simulink model "TrajectoryControl"  (R2022b)
settings: Solver=FixedStepAuto  StartTime=0.0  StopTime=30  FixedStep=0.001  RelTol=1e-3
undefined symbols (not defined in the file): h, headingangle, km, m, s, smiData, X, x, Y, Z
libraries: sm_lib x213, aerolibconvert2 x17, simulink_extras x15, nesl_utility x14, autolibshared x3, slpidlib x1, vehdynlibsteering x1, autolibutils x1
(part 1 of 5)
settings Model: Creator=dangm  LastModifiedBy=ASUS
settings SolverCC: ZeroCrossAlgorithm=Adaptive  AlgebraicLoopSolver=LineSearch
settings DebuggingCC: IgnoredZcDiagnostic=none  UnconnectedInputMsg=warning  UnconnectedOutputMsg=warning  UnconnectedLineMsg=warning  SFMachineParentedDataDiag=warning
settings ModelReferenceCC: EnableRefExpFcnMdlSchedulingChecks=on
settings ExplorerConfigSet: InternalSimMechanicsExplorerSettings="<ExplorerConfiguration><canonicalview>planar_xy</canonicalview><AnimationSetting><BasePlaybackSpeed>1.0</BasePlaybackSpeed><PlaybackSpeedFactor>1.0</PlaybackSpeedFactor></AnimationSetting><TilePanel><TileInfo><Tiles Columns=\"1\" Count=\"1\" Rows=\"1\"><Column Weight=\"1\"/><Row Weight=\"1\"/><Tile Height=\"1\" Width=\"1\" X=\"0\" Y=\"0\"/></Tiles></TileInfo><SceneInfo><SceneViewer><BGColor><R>0.60000002384185791</R><G>0.60000002384185791</G><B>0.60000002384185791</B></BGColor><Camera><DoPerspective>off</DoPerspective><Position><X>1.38151927744802361</X><Y>-0.113937833645223696</Y><Z>-0.183681847979671575</Z></Position><Center><X>0.0576620377884289326</X><Y>0.060665039066758325</Y><Z>0.733764197719871003</Z></Center><Up><X>0.27535581417737931</X><Y>0.936019488942585909</Y><Z>0.219195556338108416</Z></Up><ViewLimDist>1</ViewLimDist><YLim>0.747285369634628327</YLim><XLim>1.35610315607225207</XLim></Camera></SceneViewer></SceneInfo></TilePanel><MechEditorPanel><Cameras/><GfxPanelCameraMap/><VideoCreator><PlaybackSpeedRatio>1.0</PlaybackSpeedRatio><FrameRate>30</FrameRate><VideoFormat>Motion JPEG AVI</VideoFormat><FrameSize>auto</FrameSize></VideoCreator></MechEditorPanel></ExplorerConfiguration>"

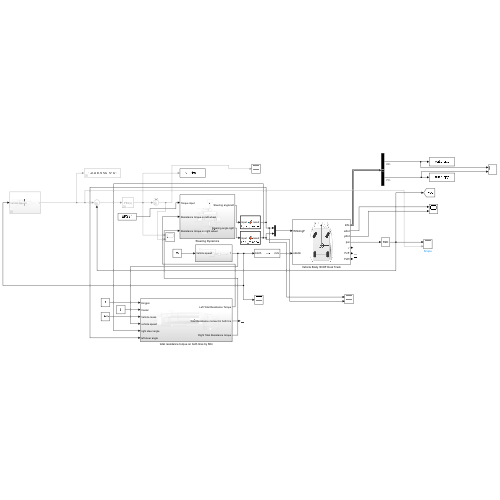
[thumbnail: Simulink's stored preview of the top-level diagram]
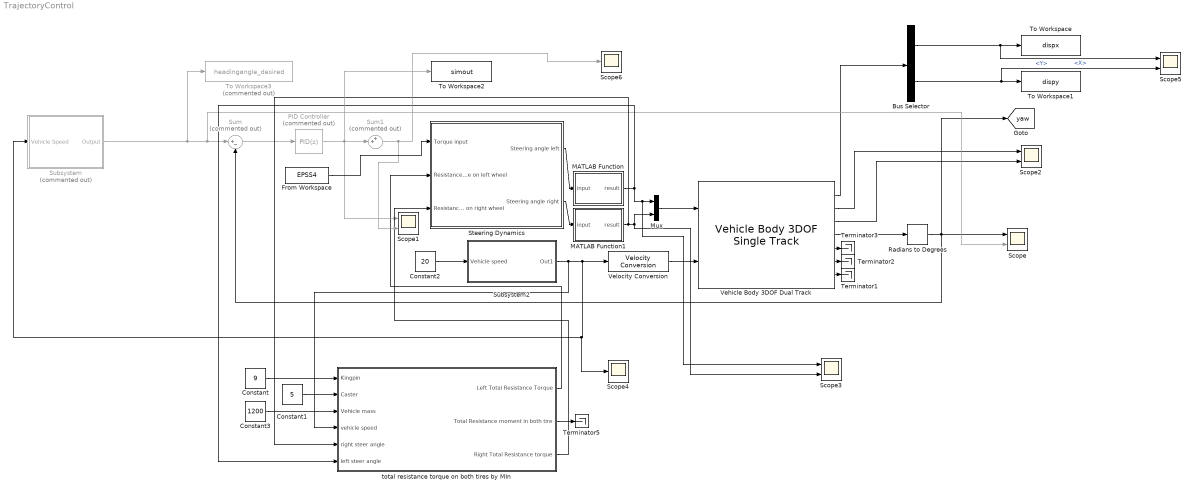
== system TrajectoryControl ==
  Bus Selector : BusSelector  OutputSignals=InertFrm.Cg.Disp.X,InertFrm.Cg.Disp.Y
  Constant : Constant  Value=9
  Constant1 : Constant  Value=5
  Constant2 : Constant  Value=20
  Constant3 : Constant  Value=1200
  From Workspace : FromWorkspace  VariableName=EPSS4
  MATLAB Function : MATLAB Function  TreatAsAtomicUnit=on
  MATLAB Function1 : MATLAB Function  TreatAsAtomicUnit=on
  Mux : Mux  Inputs=2
  PID Controller : slpidlib/PID Controller  Commented=on  Controller=PID  Form=Parallel  TimeDomain=Discrete-time  UseExternalTs=off  SampleTime=-1  IntegratorMethod=Forward Euler  FilterMethod=Forward Euler  ControllerParametersSource=internal  P=1  I=0  UseKiTs=off  D=20  N=205.123568338568  UseFilter=off  TunerSelectOption=Transfer Function Based (PID Tuner App)  InitialConditionSource=internal  InitialConditionForIntegrator=0  InitialConditionForFilter=0  DifferentiatorICPrevScaledInput=0  ExternalReset=none  TrackingMode=off  Kt=1  LimitOutput=off  SatLimitsSource=internal  UpperSaturationLimit=0  LowerSaturationLimit=-10  LinearizeAsGain=on  AntiWindupMode=none  Kb=1  LimitIntegrator=off  UpperIntegratorSaturationLimit=inf  LowerIntegratorSaturationLimit=-inf  POutMin=[]  POutMax=[]  IOutMin=[]  IOutMax=[]  DOutMin=[]  DOutMax=[]  NOutMin=[]  NOutMax=[]  SumOutMin=[]  SumOutMax=[]  SaturationOutMin=[]  SaturationOutMax=[]  PParamMin=[]  PParamMax=[]  IParamMin=[]  IParamMax=[]  DParamMin=[]  DParamMax=[]  NParamMin=[]  NParamMax=[]  KbParamMin=[]  KbParamMax=[]  KtParamMin=[]  KtParamMax=[]  KbOutMin=[]  KbOutMax=[]  KtOutMin=[]  KtOutMax=[]  IntegratorOutMin=[]  IntegratorOutMax=[]  FilterOutMin=[]  FilterOutMax=[]  SumI1OutMin=[]  SumI1OutMax=[]  SumI2OutMin=[]  SumI2OutMax=[]  SumI3OutMin=[]  SumI3OutMax=[]  SumI4OutMin=[]  SumI4OutMax=[]  SumDOutMin=[]  SumDOutMax=[]  DifferentiatorOutMin=[]  DifferentiatorOutMax=[]  FilterDiffOutCoefMin=[]  FilterDiffOutCoefMax=[]  ReciprocalOutMin=[]  ReciprocalOutMax=[]  SumDenOutMin=[]  SumDenOutMax=[]  SumNumOutMin=[]  SumNumOutMax=[]  DivideOutMin=[]  DivideOutMax=[]  UdiffTsProdOutMin=[]  UdiffTsProdOutMax=[]  NTsProdOutMin=[]  NTsProdOutMax=[]  UintegralTsProdOutMin=[]  UintegralTsProdOutMax=[]  UngainTsProdOutMin=[]  UngainTsProdOutMax=[]  ClampingZeroOutDataTypeStr=Inherit: Inherit via back propagation  ClampingZeroOutMin=[]  ClampingZeroOutMax=[]  FilterDenConstantOutDataTypeStr=Inherit: Inherit via back propagation  FilterDenConstantOutMin=[]  FilterDenConstantOutMax=[]  PCopyOutDataTypeStr=Inherit: Inherit via back propagation  PCopyOutMin=[]  PCopyOutMax=[]  NCopyOutDataTypeStr=Inherit: Inherit via back propagation  NCopyOutMin=[]  NCopyOutMax=[]  IntegratorContinuousStateAttributes=''  IntegratorStateMustResolveToSignalObject=off  IntegratorRTWStateStorageClass=Auto  FilterContinuousStateAttributes=''  FilterStateMustResolveToSignalObject=off  FilterRTWStateStorageClass=Auto  ParallelPVariant=InternalParameters  IdealPVariant=Disabled  IVariant=InternalParameters  DVariant=InternalParameters  IntegratorVariant=Discrete  SatVariant=Disabled  AWVariant=Passthrough  PCopyVariant=Disabled  TRVariant=Disabled  FdbkBlocksVariant=Forward  IdealPFdbkVariant=Disabled  SatFdbkVariant=Disabled  DerivativeFilterVariant=Differentiator  NVariant=Passthrough  NCopyVariant=Disabled_SignalSpec  FilterICVariant=InternalICsDifferentiator  IntegratorICVariant=InternalICs  ExternalResetVariant=Disabled  TRSumVariant=Passthrough  SumFdbkVariant=Disabled  SumVariant=Sum_PID  TsampFilterVariant=InternalTs  TsampNgainVariant=Passthrough  TsampIntegralVariant=Passthrough  ExternalSaturationOutDataTypeStr=Inherit: Same as second input
  Radians to Degrees : simulink_extras/Transformations/Radians to Degrees
  Scope{,1..3,5} (5 alike) : Scope  NumInputPorts=2
  Scope4 : Scope
  Scope6 : Scope
  Steering Dynamics : Subsystem
  Subsystem : Subsystem  Commented=on
  Subsystem2 : Subsystem
  Sum : Sum  Commented=on  Inputs=|+-
  Sum1 : Sum  Commented=on  Inputs=++|
  Terminator{1..3,5} (4 alike) : Terminator
  To Workspace : ToWorkspace  VariableName=dispx  SaveFormat=Structure With Time  SampleTime=-1
  To Workspace1 : ToWorkspace  VariableName=dispy  SaveFormat=Structure With Time  SampleTime=-1
  To Workspace2 : ToWorkspace  VariableName=simout  SaveFormat=Structure With Time  SampleTime=-1
  To Workspace3 : ToWorkspace  Commented=on  VariableName=headingangle_desired  SaveFormat=Structure With Time  SampleTime=-1
  Vehicle Body 3DOF Dual Track : autolibshared/Vehicle Body 3DOF Single Track  trackMode=Dual  inputMode=External longitudinal velocity  frontSteerMode=on  rearSteerMode=off  windMode=off  muMode=off  extFMode=off  extMMode=off  htchFMode=off  htchMMode=off  extXo=off  extpsio=off  extxdoto=off  extro=off  extYo=off  extTamb=off  extydoto=off  aMode=2  NF=2  NR=2  m=2000  a=1.4  b=1.6  h=0.35  dh=1  hh=0.2  X_o=0  xdot_o=0  CalphaMode=off  sigmaMode=on  d=0  hl=0  w=[1.4,1.4]  Cy_f=12e3  Cy_r=11e3  sigma_f=.1  sigma_r=.1  alpha_f_brk=[-.1 .1]  Cy_f_data=[-9e3 9e3]  alpha_r_brk=[-.1 .1]  Cy_r_data=[-9e3 9e3]  Y_o=0  ydot_o=0  Izz=4000  psi_o=0  r_o=0  Af=2  Cd=.3  Cl=.1  Cpm=.1  beta_w=[0:0.01:0.3]  Cs=[0:0.03:0.9]  Cym=[0:0.01:0.3]  Pabs=101325  Tair=273  g=9.81  mu=1  xdot_tol=.01  Fznom=5000  Fxtire_sat=7e4  Fytire_sat=7e4  longOff=0  latOff=0  vertOff=0  wrapAng=off
  Velocity Conversion : aerolibconvert2/Velocity Conversion  IU=km/h  OU=m/s
  total resistance torque on both tires by MIn : Subsystem
  tag scope: yaw=global
  wires:
  Mux/1 -> Vehicle Body 3DOF Dual Track/1
  Vehicle Body 3DOF Dual Track/7 -> Terminator1/1
  Vehicle Body 3DOF Dual Track/6 -> Terminator2/1
  Vehicle Body 3DOF Dual Track/5 -> Terminator3/1
  Vehicle Body 3DOF Dual Track/1 -> Bus Selector/1
  Vehicle Body 3DOF Dual Track/3 -> Scope2/2
  Vehicle Body 3DOF Dual Track/4 -> Radians to Degrees/1
  Radians to Degrees/1 -> [yaw], Scope/1, Sum/2
  Bus Selector/1 -> Scope5/1, To Workspace/1  "<X>"
  Bus Selector/2 -> Scope5/2, To Workspace1/1  "<Y>"
  Velocity Conversion/1 -> Vehicle Body 3DOF Dual Track/2
  Vehicle Body 3DOF Dual Track/2 -> Scope2/1
  Sum/1 -> PID Controller/1
  total resistance torque on both tires by MIn/1(Left Total Resistance Torque) -> Steering Dynamics/2(Resistance torque on left wheel)
  Subsystem2/1(Out1) -> total resistance torque on both tires by MIn/4("vehicle speed "), Scope4/1, Subsystem/1("Vehicle Speed "), Velocity Conversion/1
  Constant2/1 -> Subsystem2/1(Vehicle speed)
  Subsystem/1(Output) -> To Workspace3/1, Scope/2, Sum/1
  Steering Dynamics/1(Steering angle left) -> MATLAB Function/1(input)
  MATLAB Function/1(result) -> total resistance torque on both tires by MIn/6(left steer angle), Scope3/1, Mux/1
  Steering Dynamics/2(Steering angle right) -> MATLAB Function1/1(input)
  MATLAB Function1/1(result) -> total resistance torque on both tires by MIn/5(right steer angle), Mux/2, Scope3/2
  PID Controller/1 -> Sum1/2, To Workspace2/1, Scope1/1
  total resistance torque on both tires by MIn/3(Right Total Resistance torque) -> Steering Dynamics/3(Resistance torque on right wheel)
  total resistance torque on both tires by MIn/2(Total Resistance moment in both tire) -> Terminator5/1
  Constant/1 -> total resistance torque on both tires by MIn/1(Kingpin)
  Constant1/1 -> total resistance torque on both tires by MIn/2(Caster)
  Constant3/1 -> total resistance torque on both tires by MIn/3(Vehicle mass)
  Sum1/1 -> Scope1/2, Scope6/1
  From Workspace/1 -> Steering Dynamics/1(Torque input)

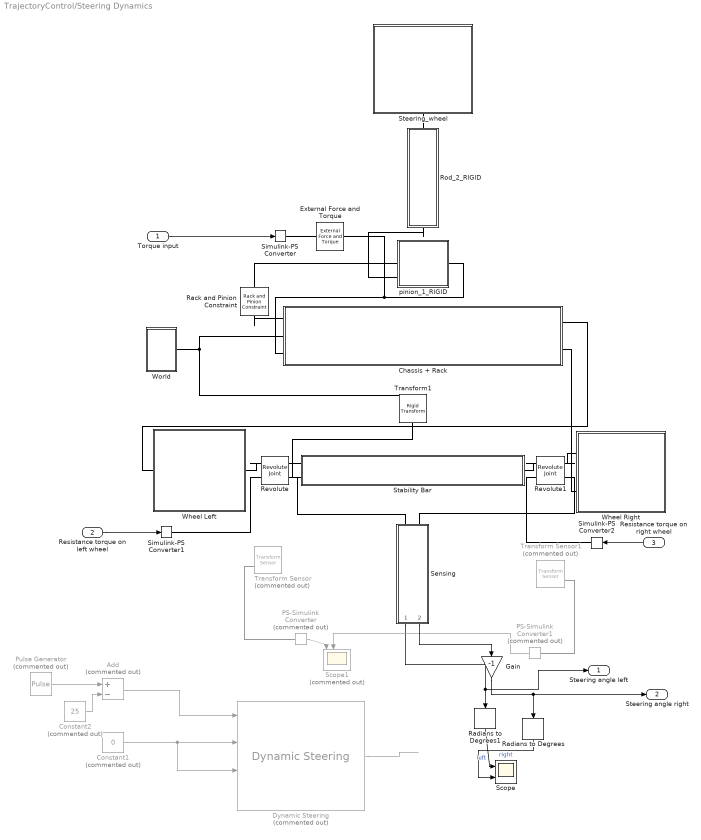
== system TrajectoryControl/Steering Dynamics ==
  Torque input : Inport
  Resistance torque on left wheel : Inport  Port=2
  Resistance torque on right wheel : Inport  Port=3
  Add : Sum  Commented=on  Inputs=+-
  Chassis + Rack : Subsystem
      mask Display: image('E:\Hoc\do an\(final) download\test14\image\Chassis+rack.png'); % Use "Edit Image" on toolstrip to change.
  Constant1 : Constant  Commented=on  Value=0
  Constant2 : Constant  Commented=on  Value=25
  Dynamic Steering : vehdynlibsteering/Dynamic Steering  Commented=on  StrgType=Rack and pinion  StrgRatioType=Constant  PwrAst=off  Loc=Front  TrckWdth=1  WhlBase=1.524  StrgRng=1.25*pi  StrgAngBpts="[-6.2832   -5.0265   -3.7699   -2.5133   -1.2566         0    1.2566    2.5133    3.7699    5.0265    6.2832]"  StrgRatioTbl=|  StrgRatio=13.5  StrgArmLngth=0.1  RckCsLngth=0.5  TieRodLngth=0.248  D=0.2  PnnRadiusTbl="[0.0055    0.0055    0.0056    0.0057    0.0057    0.0057    0.0058    0.0057    0.0056    0.0055    0.0055]"  PnnRadius=0.0057  RodLngth=0.1  ParaArmLngth=0.9  J1=0.1  J2=0.01  beta_u=0.1  beta_l=0.1  b1=0.001  k1=30  b2=1  b3=0.001  theta_o=0  omega_o=0  FricTrq=0  TrqBpts=[-100 0 100]  VehSpdBpts=[0 20]  TrqTbl=[0 -100;0 0;0 100]  TrqLmt=100  PwrLmt=1000  Eta=1  omega_c=200  aMode=2
      | [13.5000   13.3750   13.2500   13.1250   13.0000   13.0000   13.0000   13.1250   13.2500   13.3750   13.5000
      | ]
  External Force and Torque : sm_lib/Forces and Torques/External Force and Torque  ForceResolutionFrame=AttachedFrame  EnableForceX=off  EnableForceY=off  EnableForceZ=off  EnableForce=off  TorqueResolutionFrame=AttachedFrame  EnableTorqueX=off  EnableTorqueY=off  EnableTorqueZ=on  EnableTorque=off
  Gain : Gain  Gain=-1
  PS-Simulink Converter : nesl_utility/PS-Simulink Converter  Commented=on  PhysicalDomain=network_engine_domain  SubClassName=ps_output  LeftPortType=input  RightPortType=output  PseudoPeriodic=off  Frequencies=[]  VectorFormat=1-D array  Unit=inherit  AffineConversion=off
  PS-Simulink Converter1 : nesl_utility/PS-Simulink Converter  Commented=on  PhysicalDomain=network_engine_domain  SubClassName=ps_output  LeftPortType=input  RightPortType=output  PseudoPeriodic=off  Frequencies=[]  VectorFormat=1-D array  Unit=inherit  AffineConversion=off
  Pulse Generator : DiscretePulseGenerator  Commented=on  PulseType=Time based  Amplitude=50  Period=10  PulseWidth=50
  Rack and Pinion Constraint : sm_lib/Gears and Couplings/Gears/Rack and Pinion Constraint  PinionRadius=30  PinionRadiusUnits=mm
  Radians to Degrees : simulink_extras/Transformations/Radians to Degrees
  Radians to Degrees1 : simulink_extras/Transformations/Radians to Degrees
  Revolute : sm_lib/Joints/Revolute Joint  JointMode=Normal  SenseConstraintForce=off  SenseConstraintForceX=off  SenseConstraintForceY=off  SenseConstraintForceZ=off  SenseConstraintTorque=off  SenseConstraintTorqueX=off  SenseConstraintTorqueY=off  SenseConstraintTorqueZ=off  SenseTotalForce=off  SenseTotalForceX=off  SenseTotalForceY=off  SenseTotalForceZ=off  SenseTotalTorque=off  SenseTotalTorqueX=off  SenseTotalTorqueY=off  SenseTotalTorqueZ=off  CompositeWrenchDir=FollowerOnBase  CompositeWrenchFrame=BaseFrame  EquilibriumPosition=0  EquilibriumPositionUnits=deg  SpringStiffness=0.0524  SpringStiffnessUnits=N*m/deg  DampingCoefficient=1.5  DampingCoefficientUnits=N*m/(deg/s)  TorqueActuationMode=InputTorque  MotionActuationMode=ComputedMotion  SensePosition=on  SenseVelocity=off  SenseAcceleration=off  SenseTorqueForce=off  SenseLowerLimitTorqueForce=off  SenseUpperLimitTorqueForce=off  LowerLimitSpecify=on  LowerLimitBound=-2  LowerLimitBoundUnits=rad  LowerLimitStiffness=1e4  LowerLimitStiffnessUnits=N*m/deg  LowerLimitDamping=100  LowerLimitDampingUnits=N*m/(deg/s)  LowerLimitTransitionRegionWidth=0.1  LowerLimitTransitionRegionWidthUnits=deg  UpperLimitSpecify=on  UpperLimitBound=-1  UpperLimitBoundUnits=rad  UpperLimitStiffness=1e4  UpperLimitStiffnessUnits=N*m/deg  UpperLimitDamping=100  UpperLimitDampingUnits=N*m/(deg/s)  UpperLimitTransitionRegionWidth=0.1  UpperLimitTransitionRegionWidthUnits=deg  PositionTargetSpecify=on  PositionTargetPriority=High  PositionTargetValue=-89.678329494  PositionTargetValueUnits=deg  VelocityTargetSpecify=on  VelocityTargetPriority=High  VelocityTargetValue=0  VelocityTargetValueUnits=deg/s
  Revolute1 : sm_lib/Joints/Revolute Joint  JointMode=Normal  SenseConstraintForce=off  SenseConstraintForceX=off  SenseConstraintForceY=off  SenseConstraintForceZ=off  SenseConstraintTorque=off  SenseConstraintTorqueX=off  SenseConstraintTorqueY=off  SenseConstraintTorqueZ=off  SenseTotalForce=off  SenseTotalForceX=off  SenseTotalForceY=off  SenseTotalForceZ=off  SenseTotalTorque=off  SenseTotalTorqueX=off  SenseTotalTorqueY=off  SenseTotalTorqueZ=off  CompositeWrenchDir=FollowerOnBase  CompositeWrenchFrame=BaseFrame  EquilibriumPosition=0  EquilibriumPositionUnits=deg  SpringStiffness=0.0524  SpringStiffnessUnits=N*m/deg  DampingCoefficient=1.5  DampingCoefficientUnits=N*m/(deg/s)  TorqueActuationMode=InputTorque  MotionActuationMode=ComputedMotion  SensePosition=on  SenseVelocity=off  SenseAcceleration=off  SenseTorqueForce=off  SenseLowerLimitTorqueForce=off  SenseUpperLimitTorqueForce=off  LowerLimitSpecify=on  LowerLimitBound=-2  LowerLimitBoundUnits=rad  LowerLimitStiffness=1e4  LowerLimitStiffnessUnits=N*m/deg  LowerLimitDamping=100  LowerLimitDampingUnits=N*m/(deg/s)  LowerLimitTransitionRegionWidth=0.1  LowerLimitTransitionRegionWidthUnits=deg  UpperLimitSpecify=on  UpperLimitBound=-1  UpperLimitBoundUnits=rad  UpperLimitStiffness=1e4  UpperLimitStiffnessUnits=N*m/deg  UpperLimitDamping=100  UpperLimitDampingUnits=N*m/(deg/s)  UpperLimitTransitionRegionWidth=0.1  UpperLimitTransitionRegionWidthUnits=deg  PositionTargetSpecify=on  PositionTargetPriority=Low  PositionTargetValue=smiData.RevoluteJoint(2).Rz.Pos-2.7  PositionTargetValueUnits=deg  VelocityTargetSpecify=on  VelocityTargetPriority=High  VelocityTargetValue=0  VelocityTargetValueUnits=deg/s
  Rod_2_RIGID : Subsystem
      mask Display: image('rod.png'); % Use "Edit Image" on toolstrip to change.
  Scope : Scope  NumInputPorts=2
  Scope1 : Scope  Commented=on  NumInputPorts=4
  "Sensing " : Subsystem
  Simulink-PS Converter : nesl_utility/Simulink-PS Converter  PhysicalDomain=network_engine_domain  SubClassName=ps_input  LeftPortType=input  RightPortType=output  PseudoPeriodic=off  Frequencies=[]  NoiseDistribution=none  NoiseParameters=[]  Unit=N*m  AffineConversion=off  FilteringAndDerivatives=provide  SimscapeFilterOrder=1  InputFilterTimeConstant=0.001  UdotUserProvided=0
  Simulink-PS Converter1 : nesl_utility/Simulink-PS Converter  PhysicalDomain=network_engine_domain  SubClassName=ps_input  LeftPortType=input  RightPortType=output  PseudoPeriodic=off  Frequencies=[]  NoiseDistribution=none  NoiseParameters=[]  Unit=N*m  AffineConversion=off  FilteringAndDerivatives=provide  SimscapeFilterOrder=1  InputFilterTimeConstant=0.001  UdotUserProvided=0
  Simulink-PS Converter2 : nesl_utility/Simulink-PS Converter  PhysicalDomain=network_engine_domain  SubClassName=ps_input  LeftPortType=input  RightPortType=output  PseudoPeriodic=off  Frequencies=[]  NoiseDistribution=none  NoiseParameters=[]  Unit=N*m  AffineConversion=off  FilteringAndDerivatives=provide  SimscapeFilterOrder=2  InputFilterTimeConstant=0.001  UdotUserProvided=0
  Stability Bar : Subsystem
      mask Display: image('E:\Hoc\do an\(final) download\test14\image\stability bar.png'); % Use "Edit Image" on toolstrip to change.
  Steering_wheel : Subsystem
      mask Display: image('$imagefile'); % Use "Edit Image" on toolstrip to change.
  Transform Sensor : sm_lib/Frames and Transforms/Transform Sensor  Commented=on  MeasurementFrame=Base  SenseAngle=on  SenseAxis=off  SenseQ=off  SenseR=off  SenseRotationSequence=off  RotationSequence=XYX  SenseOmegaX=off  SenseOmegaY=off  SenseOmegaZ=off  SenseQDot=off  SenseRDot=off  SenseAlphaX=off  SenseAlphaY=off  SenseAlphaZ=off  SenseQDDot=off  SenseRDDot=off  SenseX=off  SenseY=off  SenseZ=off  SenseRad=off  SenseAzim=off  SenseDist=off  SenseInc=off  SenseXDot=off  SenseYDot=off  SenseZDot=off  SenseRadDot=off  SenseAzimDot=off  SenseDistDot=off  SenseIncDot=off  SenseXDDot=off  SenseYDDot=off  SenseZDDot=off  SenseRadDDot=off  SenseAzimDDot=off  SenseDistDDot=off  SenseIncDDot=off
  Transform Sensor1 : sm_lib/Frames and Transforms/Transform Sensor  Commented=on  MeasurementFrame=Base  SenseAngle=on  SenseAxis=off  SenseQ=off  SenseR=off  SenseRotationSequence=off  RotationSequence=XYX  SenseOmegaX=off  SenseOmegaY=off  SenseOmegaZ=off  SenseQDot=off  SenseRDot=off  SenseAlphaX=off  SenseAlphaY=off  SenseAlphaZ=off  SenseQDDot=off  SenseRDDot=off  SenseX=off  SenseY=off  SenseZ=off  SenseRad=off  SenseAzim=off  SenseDist=off  SenseInc=off  SenseXDot=off  SenseYDot=off  SenseZDot=off  SenseRadDot=off  SenseAzimDot=off  SenseDistDot=off  SenseIncDot=off  SenseXDDot=off  SenseYDDot=off  SenseZDDot=off  SenseRadDDot=off  SenseAzimDDot=off  SenseDistDDot=off  SenseIncDDot=off
  Transform1 : sm_lib/Frames and Transforms/Rigid Transform  TranslationMethod=Cartesian  TranslationStandardOffset=0  TranslationLengthUnit=mm  TranslationStandardAxis=+Z  TranslationCartesianOffset=smiData.RigidTransform(48).translation  TranslationROffset=0  TranslationROffsetUnits=m  TranslationZOffset=0  TranslationZOffsetUnits=m  TranslationThetaOffset=0  TranslationThetaOffsetUnits=deg  RotationMethod=ArbitraryAxis  RotationAngleUnits=rad  RotationStandardAxis=+Z  RotationAngle=smiData.RigidTransform(48).angle  RotationArbitraryAxis=smiData.RigidTransform(48).axis  FollAlignAxisA=+X  BaseAlignAxisA=+Y  FollAlignAxisB=+Y  BaseAlignAxisB=+Z  RotationSequenceAxes=FollowerAxes  RotationSequence=XYX  RotationSequenceAngles=[0 0 0]  RotationSequenceAnglesUnits=deg  RotationMatrix=[1 0 0; 0 1 0; 0 0 1]  Quaternion=[1 0 0 0]
  Wheel Left : Subsystem
      mask Display: image('E:\Hoc\do an\(final) download\test14\image\wheel.png'); % Use "Edit Image" on toolstrip to change.
  Wheel Right : Subsystem
      mask Display: image('E:\Hoc\do an\(final) download\test14\image\wheel.png'); % Use "Edit Image" on toolstrip to change.
  World : Subsystem
  pinion_1_RIGID : Subsystem
      mask Display: image('pinion.png'); % Use "Edit Image" on toolstrip to change.
  Steering angle left : Outport
  Steering angle right : Outport  Port=2
  wires:
  "Sensing "/1(Steering angle left (rad)) -> Steering angle left/1, Radians to Degrees1/1
  Add/1 -> Dynamic Steering/1
  Pulse Generator/1 -> Add/1
  Gain/1 -> Steering angle right/1, Radians to Degrees/1
  PS-Simulink Converter1/1 -> Scope1/2
  Constant2/1 -> Add/2
  Constant1/1 -> Dynamic Steering/3, Dynamic Steering/2
  Dynamic Steering/2 -> ?
  "Sensing "/2(Steering angle right (rad)) -> Gain/1
  PS-Simulink Converter/1 -> Scope1/1
  Torque input/1 -> Simulink-PS Converter/1
  Resistance torque on left wheel/1 -> Simulink-PS Converter1/1
  Resistance torque on right wheel/1 -> Simulink-PS Converter2/1
  Radians to Degrees/1 -> Scope/2  "right"
  Radians to Degrees1/1 -> Scope/1  "left"
  connections:
  PS-Simulink Converter1/LConn1 -- Transform Sensor1/RConn2
  Revolute/RConn2 -- "Sensing "/LConn1
  Simulink-PS Converter/RConn1 -- External Force and Torque/LConn1
  Chassis + Rack/LConn2 -- World/LConn1 -- Transform1/LConn1
  Rack and Pinion Constraint/RConn1 -- Chassis + Rack/LConn1
  PS-Simulink Converter/LConn1 -- Transform Sensor/RConn2
  "Sensing "/LConn2 -- Revolute1/RConn2
  Rack and Pinion Constraint/LConn1 -- pinion_1_RIGID/LConn2
  Transform1/RConn1 -- Stability Bar/LConn2
  Chassis + Rack/LConn3 -- External Force and Torque/RConn1 -- pinion_1_RIGID/RConn1
  Chassis + Rack/RConn1 -- Wheel Left/LConn1
  Revolute1/RConn1 -- Wheel Right/LConn1
  Chassis + Rack/RConn2 -- Wheel Right/LConn2
  Revolute1/LConn1 -- Stability Bar/RConn1
  Revolute/RConn1 -- Stability Bar/LConn1
  Revolute/LConn1 -- Wheel Left/RConn1
  Rod_2_RIGID/RConn1 -- pinion_1_RIGID/LConn3
  Steering_wheel/LConn1 -- Rod_2_RIGID/LConn1
  Simulink-PS Converter1/RConn1 -- Revolute/LConn2
  Simulink-PS Converter2/RConn1 -- Revolute1/LConn2

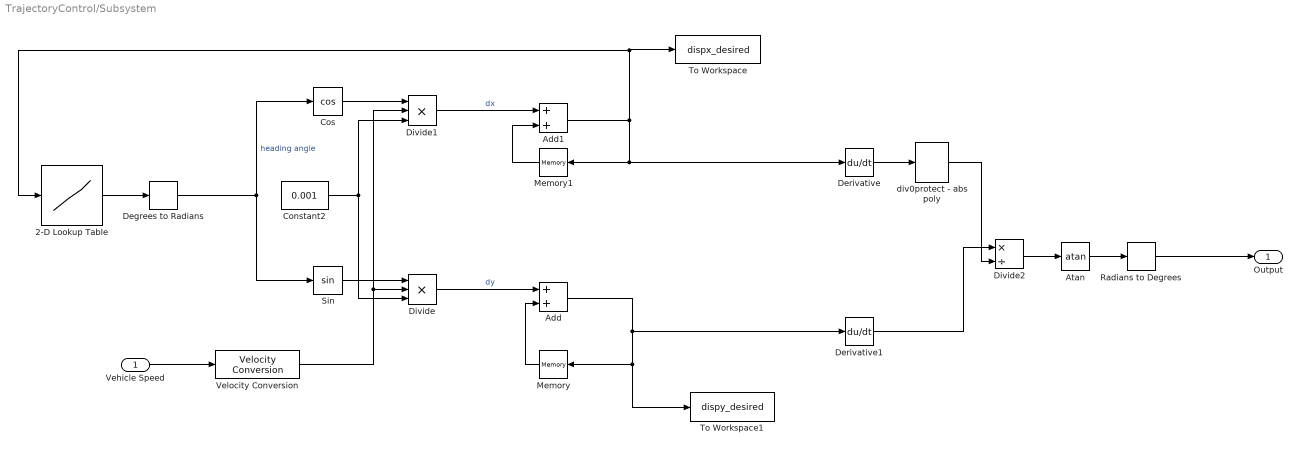
== system TrajectoryControl/Subsystem ==
  "Vehicle Speed " : Inport
  2-D Lookup Table : Lookup_n-D  NumberOfTableDimensions=1  BreakpointsForDimension1=x  BreakpointsForDimension2=[1:3]  Table=headingangle  InternalRulePriority=Speed  RndMeth=Simplest
  Add : Sum
  Add1 : Sum
  Atan : Trigonometry  Operator=atan
  Constant2 : Constant  Value=0.001
  Cos : Trigonometry  Operator=cos
  Degrees to Radians : simulink_extras/Transformations/Degrees to Radians
  Derivative : Derivative
  Derivative1 : Derivative
  Divide : Product  Inputs=***
  Divide1 : Product  Inputs=***
  Divide2 : Product  Inputs=*/
  Memory : Memory
  Memory1 : Memory
  Radians to Degrees : simulink_extras/Transformations/Radians to Degrees
  Sin : Trigonometry
  To Workspace : ToWorkspace  VariableName=dispx_desired  SaveFormat=Structure With Time  SampleTime=-1
  To Workspace1 : ToWorkspace  VariableName=dispy_desired  SaveFormat=Structure With Time  SampleTime=-1
  Velocity Conversion : aerolibconvert2/Velocity Conversion  IU=km/h  OU=m/s
  div0protect - abs poly : autolibutils/div0protect - abs poly  thresh=1e-6  aMode=aMode
  Output : Outport
  wires:
  Constant2/1 -> Divide/3, Divide1/3
  Sin/1 -> Divide/1
  Degrees to Radians/1 -> Sin/1, Cos/1  "heading angle"
  Atan/1 -> Radians to Degrees/1
  Add/1 -> Memory/1, To Workspace1/1, Derivative1/1
  "Vehicle Speed "/1 -> Velocity Conversion/1
  Velocity Conversion/1 -> Divide/2, Divide1/2
  Divide1/1 -> Add1/1  "dx"
  Derivative/1 -> div0protect - abs poly/1
  Memory/1 -> Add/2
  Add1/1 -> Memory1/1, Derivative/1, 2-D Lookup Table/1, To Workspace/1
  Cos/1 -> Divide1/1
  Derivative1/1 -> Divide2/1
  Divide2/1 -> Atan/1
  Divide/1 -> Add/1  "dy"
  Memory1/1 -> Add1/2
  2-D Lookup Table/1 -> Degrees to Radians/1
  div0protect - abs poly/1 -> Divide2/2
  Radians to Degrees/1 -> Output/1

== system TrajectoryControl/Subsystem2 ==
  Vehicle speed : Inport
  Constant : Constant  Value=10
  Switch : Switch  Criteria=u2 > Threshold  SaturateOnIntegerOverflow=off  InputSameDT=off
  Out1 : Outport
  wires:
  Switch/1 -> Out1/1
  [yaw] -> Switch/2
  Constant/1 -> Switch/1
  Vehicle speed/1 -> Switch/3

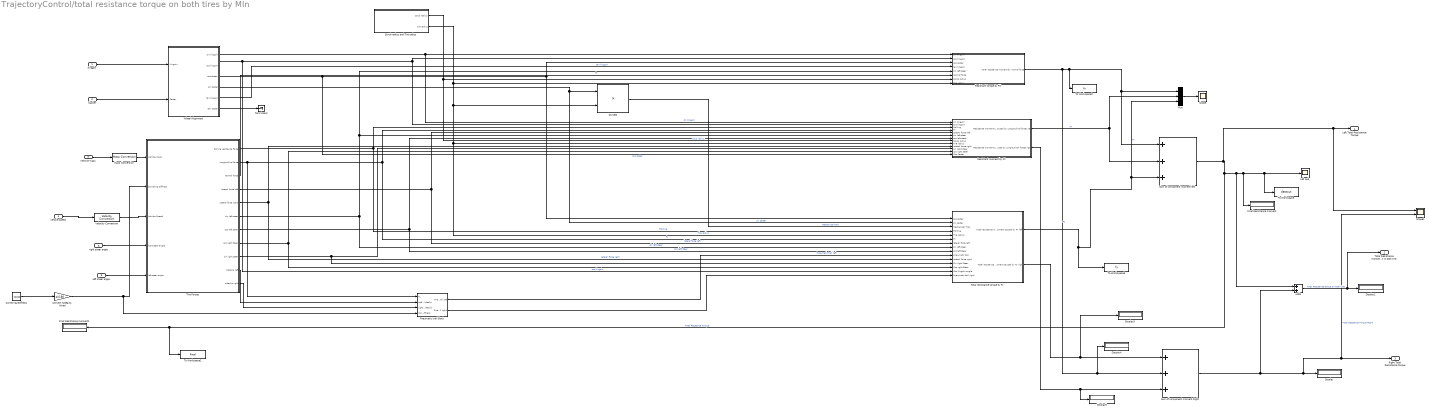
== system TrajectoryControl/total resistance torque on both tires by MIn ==
  Kingpin : Inport
  Caster : Inport  Port=2
  Vehicle mass : Inport  Port=3
  "vehicle speed " : Inport  Port=4
  right steer angle : Inport  Port=5
  left steer angle : Inport  Port=6
  Add1 : Sum
  Convert N/deg to N/rad : Gain  Gain=pi/180
  Cornering Stiffness : Constant  Value=20000
  Display{,1,3..5} (5 alike) : Display
  Divide2 : Product  Inputs=**
  Final Resistance moment : Display
  Final Resistance moment1 : Display
  Kết quả : Scope
  Mass Conversion : aerolibconvert2/Mass Conversion  IU=kg  OU=kg
  Mux : Mux  Inputs=3
  Pneumatic trail block : Subsystem
  Resistant moment by FX : Subsystem
  Resistant torque by FZ : Subsystem
  Scope : Scope
  Scope1 : Scope  NumInputPorts=2
  Scrub radius and Tire radius : Subsystem
  Sum of component moment Right : Sum  Inputs=+++
  Sum of component moment left : Sum  Inputs=+++
  Terminator : Terminator
  Tire Forces : Subsystem
  To Workspace : ToWorkspace  VariableName=dataout  SaveFormat=Timeseries  SampleTime=-1
  To Workspace1 : ToWorkspace  VariableName=final  SaveFormat=Timeseries  SampleTime=-1
  To Workspace2 : ToWorkspace  VariableName=fx  SaveFormat=Timeseries  SampleTime=-1
  To Workspace3 : ToWorkspace  VariableName=fy  SaveFormat=Timeseries  SampleTime=-1
  Total resistance torque by Fy : Subsystem
  Velocity Conversion : aerolibconvert2/Velocity Conversion  IU=km/h  OU=m/s
  Wheel Alignment : Subsystem
  Left Total Resistance Torque : Outport
  Total Resistance moment in both tire : Outport  Port=2
  Right Total Resistance torque : Outport  Port=3
  wires:
  Add1/1 -> Total Resistance moment in both tire/1, Display1/1  "Total Resistance torque on both tires"
  Resistant torque by FZ/1(Toral resistance moment by normal force) -> Display4/1, Sum of component moment Right/2, To Workspace2/1, Mux/1, Sum of component moment left/1  "Fz"
  Tire Forces/2(Longitudinal force) -> Pneumatic trail block/1(Fx), Total resistance torque by Fy/6(Fx), Resistant moment by FX/4(Fx)  "Fx"
  Sum of component moment Right/1 -> Add1/2, Scope1/2, Right Total Resistance torque/1, Display/1  "Total Resstance Torque Right"
  Kingpin/1 -> Wheel Alignment/1(Kingpin)
  Total resistance torque by Fy/1("Total resistance moment caused by FY lefft ") -> To Workspace3/1, Mux/3, Sum of component moment left/3  "Fy"
  Sum of component moment left/1 -> Scope1/1, Left Total Resistance Torque/1, To Workspace1/1, Final Resistance moment1/1, Add1/1, To Workspace/1, Kết quả/1, Final Resistance moment/1  "Total Resstance Torque"
  Wheel Alignment/6(tan caster) -> Terminator/1
  Wheel Alignment/3(cos caster) -> Resistant moment by FX/13(Cos Caster), Total resistance torque by Fy/1(cos caster), Resistant torque by FZ/3(cos caster)  "cos caster"
  Scrub radius and Tire radius/2(tire radius) -> Total resistance torque by Fy/5(Tire radius), Resistant moment by FX/9(Tire radius), Divide2/2, Resistant torque by FZ/8(Tire radius)  "Tire radius"
  Tire Forces/8(cos right steer) -> Resistant moment by FX/12(cos right steer), Total resistance torque by Fy/13(Cos right Steer)
  Vehicle mass/1 -> Mass Conversion/1
  Scrub radius and Tire radius/1(scrub radius) -> Resistant moment by FX/8(Scrub radius), Resistant torque by FZ/7(Scrub radius)  "Scub radius"
  Resistant moment by FX/1(Resistance moment caused by Longitudinal forces left) -> Sum of component moment left/2, Mux/2  "Fx"
  Wheel Alignment/1(sin kingpin) -> Resistant moment by FX/1(sin kingpin), Resistant torque by FZ/1(sin kingpin)  "sin kingpin"
  Tire Forces/7(cos left steer) -> Total resistance torque by Fy/9(cos left steer), Resistant moment by FX/7(cos left steer)  "cos left steer"
  "vehicle speed "/1 -> Velocity Conversion/1
  Wheel Alignment/4(sin caster) -> Total resistance torque by Fy/2(sin caster), Divide2/1  "sin caster"
  Mass Conversion/1 -> Tire Forces/1(vehicle mass)
  Convert N/deg to N/rad/1 -> Pneumatic trail block/4(Cornering Stiffness), Tire Forces/2(Cornering stiffness)
  Tire Forces/1(Rolling resistance Force) -> Resistant moment by FX/3(Frolling), Total resistance torque by Fy/4(Frolling)  "Frolling"
  Mux/1 -> Scope/1
  Tire Forces/6(sin left steer) -> Total resistance torque by Fy/8(sin left steer), Resistant torque by FZ/5(sin left steer), Resistant moment by FX/6(sin left steer)  "sin left steer"
  Tire Forces/4(Lateral force left) -> Total resistance torque by Fy/7(lateral force left), Resistant moment by FX/5(Lateral force left)  "lateral force left"
  Wheel Alignment/2(cos kingpin) -> Total resistance torque by Fy/14(Cos Kingpin angle), Resistant torque by FZ/2(cos kingpin), Resistant moment by FX/2(cos kingpin)  "cos kingpin"
  Tire Forces/10(sidelsip left) -> Pneumatic trail block/2(Left sideslip)
  Tire Forces/11(sideslip right) -> Pneumatic trail block/3(right sideslip)
  Cornering Stiffness/1 -> Convert N/deg to N/rad/1
  Tire Forces/3(Normal force) -> Resistant torque by FZ/6(Normal force)  "Fz"
  Divide2/1 -> Total resistance torque by Fy/3(Mechanical Trail)  "Mechanical Trail"
  Wheel Alignment/5(tan kingpin) -> Resistant torque by FZ/4(tan kingpin)  "tan kingpin"
  Pneumatic trail block/1(Pneumatic Trail left) -> Total resistance torque by Fy/10(pneumatic trail)  "Pneumatic trail left"
  Tire Forces/5(Lateral force right) -> Resistant moment by FX/10(Lateral force right), Total resistance torque by Fy/11(Lateral Force right)  "Lateral Force right"
  Tire Forces/9(sin right steer) -> Resistant moment by FX/11(sin right steer), Total resistance torque by Fy/12(Sin right Steer)
  Total resistance torque by Fy/2(Total resistance moment caused by Fy right) -> Display3/1, Sum of component moment Right/1
  Caster/1 -> Wheel Alignment/2(Caster)
  Resistant moment by FX/2(Resistance moment caused by Longitudinal forces right) -> Display5/1, Sum of component moment Right/3
  Velocity Conversion/1 -> Tire Forces/3(Vehicle Speed)
  Pneumatic trail block/2(Pneumatic Trail right) -> Total resistance torque by Fy/15(Pneumatic trail right)
  right steer angle/1 -> Tire Forces/4("right steer angle ")
  left steer angle/1 -> Tire Forces/5("left steer angle ")

== system TrajectoryControl/Steering Dynamics/Chassis + Rack ==
  Rack Case + Chassis : Subsystem
  Rack_1_RIGID : Subsystem
  Target : PMIOPort  Side=Left
  Conn3 : PMIOPort  Port=2  Side=Left
  Conn1 : PMIOPort  Port=3  Side=Left
  F2 : PMIOPort  Port=4  Side=Right
  F3 : PMIOPort  Port=5  Side=Right
  connections:
  Rack_1_RIGID/RConn1 -- Rack Case + Chassis/LConn2
  Rack_1_RIGID/RConn2 -- Rack Case + Chassis/LConn3
  Rack_1_RIGID/RConn4 -- Rack Case + Chassis/LConn5
  Conn3/RConn1 -- Rack Case + Chassis/LConn1
  Target/RConn1 -- Rack_1_RIGID/LConn1
  Rack Case + Chassis/LConn4 -- Rack_1_RIGID/RConn3
  Rack Case + Chassis/LConn7 -- F2/RConn1
  Rack Case + Chassis/LConn6 -- Rack_1_RIGID/RConn5
  Rack Case + Chassis/RConn2 -- F3/RConn1
  Rack Case + Chassis/RConn1 -- Conn1/RConn1

== system TrajectoryControl/Steering Dynamics/Rod_2_RIGID ==
  ReferenceFrame : sm_lib/Frames and Transforms/Reference Frame
  Solid : sm_lib/Body Elements/File Solid  ExtGeomFileName=Rod_Default_sldprt.STEP  UnitType=FromFile  ExtGeomFileUnits=m  StepReaderType=HEX  ExportConvexHullGeometry=off  InertiaType=Custom  Mass=smiData.Solid(4).mass  MassUnits=kg  CenterOfMass=smiData.Solid(4).CoM  CenterOfMassUnits=mm  MomentsOfInertia=smiData.Solid(4).MoI  MomentsOfInertiaUnits=kg*mm^2  ProductsOfInertia=smiData.Solid(4).PoI  ProductsOfInertiaUnits=kg*mm^2  BasedOnType=DensityFromFile  Density=1000  DensityUnits=kg/m^3  DoExposeReferenceFrame=on  SerializedFrames=<Frames/>  GraphicType=FromGeometry  MarkerShape=Sphere  MarkerSize=10  GraphicVisPropType=SimpleVisualProperties  GraphicDiffuseColor=smiData.Solid(4).color  GraphicSpecularColor=[0.5 0.5 0.5 1.0]  GraphicAmbientColor=[0.15 0.15 0.15 1.0]  GraphicEmissiveColor=[0.0 0.0 0.0 1.0]  GraphicShininess=75  GraphicOpacity=smiData.Solid(4).opacity
  Transform : sm_lib/Frames and Transforms/Rigid Transform  TranslationMethod=Cartesian  TranslationStandardOffset=0  TranslationLengthUnit=mm  TranslationStandardAxis=+Z  TranslationCartesianOffset=smiData.RigidTransform(39).translation  TranslationROffset=0  TranslationROffsetUnits=m  TranslationZOffset=0  TranslationZOffsetUnits=m  TranslationThetaOffset=0  TranslationThetaOffsetUnits=deg  RotationMethod=ArbitraryAxis  RotationAngleUnits=rad  RotationStandardAxis=+Z  RotationAngle=smiData.RigidTransform(39).angle  RotationArbitraryAxis=smiData.RigidTransform(39).axis  FollAlignAxisA=+X  BaseAlignAxisA=+Y  FollAlignAxisB=+Y  BaseAlignAxisB=+Z  RotationSequenceAxes=FollowerAxes  RotationSequence=XYX  RotationSequenceAngles=[0 0 0]  RotationSequenceAnglesUnits=deg  RotationMatrix=[1 0 0; 0 1 0; 0 0 1]  Quaternion=[1 0 0 0]
  Transform1 : sm_lib/Frames and Transforms/Rigid Transform  TranslationMethod=Cartesian  TranslationStandardOffset=0  TranslationLengthUnit=mm  TranslationStandardAxis=+Z  TranslationCartesianOffset=smiData.RigidTransform(42).translation  TranslationROffset=0  TranslationROffsetUnits=m  TranslationZOffset=0  TranslationZOffsetUnits=m  TranslationThetaOffset=0  TranslationThetaOffsetUnits=deg  RotationMethod=ArbitraryAxis  RotationAngleUnits=rad  RotationStandardAxis=+Z  RotationAngle=smiData.RigidTransform(42).angle  RotationArbitraryAxis=smiData.RigidTransform(42).axis  FollAlignAxisA=+X  BaseAlignAxisA=+Y  FollAlignAxisB=+Y  BaseAlignAxisB=+Z  RotationSequenceAxes=FollowerAxes  RotationSequence=XYX  RotationSequenceAngles=[0 0 0]  RotationSequenceAnglesUnits=deg  RotationMatrix=[1 0 0; 0 1 0; 0 0 1]  Quaternion=[1 0 0 0]
  F : PMIOPort  Side=Left
  F1 : PMIOPort  Port=2  Side=Right
  connections:
  Solid/RConn1 -- ReferenceFrame/RConn1 -- Transform/LConn1 -- Transform1/LConn1
  Transform/RConn1 -- F/RConn1
  Transform1/RConn1 -- F1/RConn1

== system TrajectoryControl/Steering Dynamics/Sensing  ==
  Add : Sum
  Add1 : Sum
  Constant1 : Constant  Value=1.5458-2.6414e-05+0.01940853136
  Constant2 : Constant  Value=1.5847-(-2.3866e-05)-0.019541748665
  PS-Simulink Converter : nesl_utility/PS-Simulink Converter  PhysicalDomain=network_engine_domain  SubClassName=ps_output  LeftPortType=input  RightPortType=output  PseudoPeriodic=off  Frequencies=[]  VectorFormat=1-D array  Unit=rad  AffineConversion=off
  PS-Simulink Converter1 : nesl_utility/PS-Simulink Converter  PhysicalDomain=network_engine_domain  SubClassName=ps_output  LeftPortType=input  RightPortType=output  PseudoPeriodic=off  Frequencies=[]  VectorFormat=1-D array  Unit=rad  AffineConversion=off
  Radians to Degrees : simulink_extras/Transformations/Radians to Degrees
  Radians to Degrees1 : simulink_extras/Transformations/Radians to Degrees
  Scope : Scope  NumInputPorts=2
  To Workspace : ToWorkspace  VariableName=left  SaveFormat=Structure  SampleTime=-1
  To Workspace1 : ToWorkspace  VariableName=right  SaveFormat=Structure  SampleTime=-1
  input : PMIOPort  Side=Left
  input1 : PMIOPort  Port=2  Side=Left
  Steering angle left (rad) : Outport
  Steering angle right (rad) : Outport  Port=2
  wires:
  Constant1/1 -> Add/2
  PS-Simulink Converter1/1 -> Radians to Degrees1/1, Add1/1, To Workspace1/1  "Steering angle right (rad)"
  PS-Simulink Converter/1 -> To Workspace/1, Radians to Degrees/1, Add/1  "Steering angle left (rad)"
  Constant2/1 -> Add1/2
  Add/1 -> Steering angle left (rad)/1  "Steering angle left (rad)"
  Add1/1 -> Steering angle right (rad)/1  "Steering angle right (rad)"
  Radians to Degrees/1 -> Scope/1  "left"
  Radians to Degrees1/1 -> Scope/2  "right"
  connections:
  input/RConn1 -- PS-Simulink Converter/LConn1
  input1/RConn1 -- PS-Simulink Converter1/LConn1

== system TrajectoryControl/Steering Dynamics/Stability Bar ==
  ReferenceFrame : sm_lib/Frames and Transforms/Reference Frame
  Solid : sm_lib/Body Elements/File Solid  ExtGeomFileName=lock_arm by Long_Default_sldprt.STEP  UnitType=FromFile  ExtGeomFileUnits=m  StepReaderType=HEX  ExportConvexHullGeometry=off  InertiaType=Custom  Mass=smiData.Solid(12).mass  MassUnits=kg  CenterOfMass=smiData.Solid(12).CoM  CenterOfMassUnits=mm  MomentsOfInertia=smiData.Solid(12).MoI  MomentsOfInertiaUnits=kg*mm^2  ProductsOfInertia=smiData.Solid(12).PoI  ProductsOfInertiaUnits=kg*mm^2  BasedOnType=DensityFromFile  Density=1000  DensityUnits=kg/m^3  DoExposeReferenceFrame=on  SerializedFrames=<Frames/>  GraphicType=FromGeometry  MarkerShape=Sphere  MarkerSize=10  GraphicVisPropType=SimpleVisualProperties  GraphicDiffuseColor=smiData.Solid(12).color  GraphicSpecularColor=[0.5 0.5 0.5 1.0]  GraphicAmbientColor=[0.15 0.15 0.15 1.0]  GraphicEmissiveColor=[0.0 0.0 0.0 1.0]  GraphicShininess=75  GraphicOpacity=smiData.Solid(12).opacity
  Transform : sm_lib/Frames and Transforms/Rigid Transform  TranslationMethod=Cartesian  TranslationStandardOffset=0  TranslationLengthUnit=mm  TranslationStandardAxis=+Z  TranslationCartesianOffset=smiData.RigidTransform(2).translation  TranslationROffset=0  TranslationROffsetUnits=m  TranslationZOffset=0  TranslationZOffsetUnits=m  TranslationThetaOffset=0  TranslationThetaOffsetUnits=deg  RotationMethod=ArbitraryAxis  RotationAngleUnits=rad  RotationStandardAxis=+Z  RotationAngle=smiData.RigidTransform(2).angle  RotationArbitraryAxis=smiData.RigidTransform(2).axis  FollAlignAxisA=+X  BaseAlignAxisA=+Y  FollAlignAxisB=+Y  BaseAlignAxisB=+Z  RotationSequenceAxes=FollowerAxes  RotationSequence=XYX  RotationSequenceAngles=[0 0 0]  RotationSequenceAnglesUnits=deg  RotationMatrix=[1 0 0; 0 1 0; 0 0 1]  Quaternion=[1 0 0 0]
  Transform1 : sm_lib/Frames and Transforms/Rigid Transform  TranslationMethod=Cartesian  TranslationStandardOffset=0  TranslationLengthUnit=mm  TranslationStandardAxis=+Z  TranslationCartesianOffset=smiData.RigidTransform(3).translation  TranslationROffset=0  TranslationROffsetUnits=m  TranslationZOffset=0  TranslationZOffsetUnits=m  TranslationThetaOffset=0  TranslationThetaOffsetUnits=deg  RotationMethod=ArbitraryAxis  RotationAngleUnits=rad  RotationStandardAxis=+Z  RotationAngle=smiData.RigidTransform(3).angle  RotationArbitraryAxis=smiData.RigidTransform(3).axis  FollAlignAxisA=+X  BaseAlignAxisA=+Y  FollAlignAxisB=+Y  BaseAlignAxisB=+Z  RotationSequenceAxes=FollowerAxes  RotationSequence=XYX  RotationSequenceAngles=[0 0 0]  RotationSequenceAnglesUnits=deg  RotationMatrix=[1 0 0; 0 1 0; 0 0 1]  Quaternion=[1 0 0 0]
  F : PMIOPort  Side=Left
  F2 : PMIOPort  Port=2  Side=Left
  F1 : PMIOPort  Port=3  Side=Right
  connections:
  Solid/RConn1 -- ReferenceFrame/RConn1 -- Transform/LConn1 -- Transform1/LConn1 -- F2/RConn1
  Transform/RConn1 -- F/RConn1
  Transform1/RConn1 -- F1/RConn1

== system TrajectoryControl/Steering Dynamics/Steering_wheel ==
  ReferenceFrame : sm_lib/Frames and Transforms/Reference Frame
  Solid : sm_lib/Body Elements/File Solid  ExtGeomFileName=Steering wheel_Default_sldprt.STEP  UnitType=FromFile  ExtGeomFileUnits=m  StepReaderType=HEX  ExportConvexHullGeometry=off  InertiaType=Custom  Mass=smiData.Solid(9).mass  MassUnits=kg  CenterOfMass=smiData.Solid(9).CoM  CenterOfMassUnits=mm  MomentsOfInertia=smiData.Solid(9).MoI  MomentsOfInertiaUnits=kg*mm^2  ProductsOfInertia=smiData.Solid(9).PoI  ProductsOfInertiaUnits=kg*mm^2  BasedOnType=DensityFromFile  Density=1000  DensityUnits=kg/m^3  DoExposeReferenceFrame=on  SerializedFrames=<Frames/>  GraphicType=FromGeometry  MarkerShape=Sphere  MarkerSize=10  GraphicVisPropType=SimpleVisualProperties  GraphicDiffuseColor=smiData.Solid(9).color  GraphicSpecularColor=[0.5 0.5 0.5 1.0]  GraphicAmbientColor=[0.15 0.15 0.15 1.0]  GraphicEmissiveColor=[0.0 0.0 0.0 1.0]  GraphicShininess=75  GraphicOpacity=smiData.Solid(9).opacity
  Transform : sm_lib/Frames and Transforms/Rigid Transform  TranslationMethod=Cartesian  TranslationStandardOffset=0  TranslationLengthUnit=mm  TranslationStandardAxis=+Z  TranslationCartesianOffset=smiData.RigidTransform(40).translation  TranslationROffset=0  TranslationROffsetUnits=m  TranslationZOffset=0  TranslationZOffsetUnits=m  TranslationThetaOffset=0  TranslationThetaOffsetUnits=deg  RotationMethod=ArbitraryAxis  RotationAngleUnits=rad  RotationStandardAxis=+Z  RotationAngle=smiData.RigidTransform(40).angle  RotationArbitraryAxis=smiData.RigidTransform(40).axis  FollAlignAxisA=+X  BaseAlignAxisA=+Y  FollAlignAxisB=+Y  BaseAlignAxisB=+Z  RotationSequenceAxes=FollowerAxes  RotationSequence=XYX  RotationSequenceAngles=[0 0 0]  RotationSequenceAnglesUnits=deg  RotationMatrix=[1 0 0; 0 1 0; 0 0 1]  Quaternion=[1 0 0 0]
  F : PMIOPort  Side=Left
  connections:
  Solid/RConn1 -- ReferenceFrame/RConn1 -- Transform/LConn1
  Transform/RConn1 -- F/RConn1

== system TrajectoryControl/Steering Dynamics/Wheel Left ==
  Innova_Crysta_Assembly_Final_1_RIGID : Subsystem
  wheelpin_by_Long_1_RIGID : Subsystem
  F2 : PMIOPort  Side=Left
  F : PMIOPort  Port=2  Side=Right
  connections:
  Innova_Crysta_Assembly_Final_1_RIGID/RConn1 -- wheelpin_by_Long_1_RIGID/LConn1
  F2/RConn1 -- wheelpin_by_Long_1_RIGID/RConn2
  F/RConn1 -- wheelpin_by_Long_1_RIGID/RConn1

== system TrajectoryControl/Steering Dynamics/Wheel Right ==
  Innova_Crysta_Assembly_Final_2_RIGID : Subsystem
  wheelpin_by_Long_2_RIGID : Subsystem
  F : PMIOPort  Side=Left
  F2 : PMIOPort  Port=2  Side=Left
  connections:
  Innova_Crysta_Assembly_Final_2_RIGID/RConn1 -- wheelpin_by_Long_2_RIGID/RConn1
  F2/RConn1 -- wheelpin_by_Long_2_RIGID/LConn2
  F/RConn1 -- wheelpin_by_Long_2_RIGID/LConn1

== system TrajectoryControl/Steering Dynamics/World ==
  MechanismConfiguration : sm_lib/Utilities/Mechanism Configuration  UniformGravity=Constant  GravityVector=[0 0 0]  GravityUnits=m/s^2  LinearizationDelta=0.001  JointModeTransitionNonlinearIterations=2
  Solver Configuration : nesl_utility/Solver Configuration  PhysicalDomain=network_engine_domain  SubClassName=solver  LeftPortType=input  RightPortType=generic  Tones=[]  Harmonics=[]  SimulateNoise=off  Profile=off  UseLocalSampling=off  EnableSwitchedLinearOptims=on  FrequencyDomain=off  UseCCode=off  RelTol=0.001  AbsTol=0.001  MinStep=1e-09  ToWorkspace=off  RevertToSquareIcSolve=off  NumHomotopyIterations=100  PhasorMode=off  PhasorModeNumHarmonics=1  ConsistencySolver=NEWTON_FTOL  IndexReductionMethod=DerivativeReplacement  DoDC=off  ResidualTolerance=1e-09  ConsistencyTolSource=GLOBAL  ConsistencyAbsTol=0.001  ConsistencyRelTol=0.001  ConsistencyTolFactor=0.001  UseLocalSolver=off  LocalSolverChoice=NE_BACKWARD_EULER_ADVANCER  ResolveIndetEquations=on  FunctionEvalNumThread=1  LocalSolverSampleTime=0.001  DoFixedCost=off  MaxNonlinIter=3  MaxModeIter=2  ComputeImpulses=off  ImpulseIterations=2  LinearAlgebra=auto  LinearAlgebraNumThread=0  EquationFormulation=NE_TIME_EF  DelaysMemoryBudget=1024  AutomaticFiltering=on  FilteringTimeConstant=0.001  PartitionStorageMethod=AS_NEEDED  PartitionMemoryBudget=1024  PartitionMethod=ROBUST
  World : sm_lib/Frames and Transforms/World Frame
  Conn1 : PMIOPort  Side=Left
  connections:
  MechanismConfiguration/RConn1 -- Conn1/RConn1 -- World/RConn1 -- Solver Configuration/RConn1

== system TrajectoryControl/Steering Dynamics/pinion_1_RIGID ==
  ReferenceFrame : sm_lib/Frames and Transforms/Reference Frame
  Solid : sm_lib/Body Elements/File Solid  ExtGeomFileName=pinion_Default_sldprt.STEP  UnitType=FromFile  ExtGeomFileUnits=m  StepReaderType=HEX  ExportConvexHullGeometry=off  InertiaType=Custom  Mass=smiData.Solid(8).mass  MassUnits=kg  CenterOfMass=smiData.Solid(8).CoM  CenterOfMassUnits=mm  MomentsOfInertia=smiData.Solid(8).MoI  MomentsOfInertiaUnits=kg*mm^2  ProductsOfInertia=smiData.Solid(8).PoI  ProductsOfInertiaUnits=kg*mm^2  BasedOnType=DensityFromFile  Density=1000  DensityUnits=kg/m^3  DoExposeReferenceFrame=on  SerializedFrames=<Frames/>  GraphicType=FromGeometry  MarkerShape=Sphere  MarkerSize=10  GraphicVisPropType=SimpleVisualProperties  GraphicDiffuseColor=smiData.Solid(8).color  GraphicSpecularColor=[0.5 0.5 0.5 1.0]  GraphicAmbientColor=[0.15 0.15 0.15 1.0]  GraphicEmissiveColor=[0.0 0.0 0.0 1.0]  GraphicShininess=75  GraphicOpacity=smiData.Solid(8).opacity
  Transform : sm_lib/Frames and Transforms/Rigid Transform  TranslationMethod=Cartesian  TranslationStandardOffset=0  TranslationLengthUnit=mm  TranslationStandardAxis=+Z  TranslationCartesianOffset=smiData.RigidTransform(12).translation  TranslationROffset=0  TranslationROffsetUnits=m  TranslationZOffset=0  TranslationZOffsetUnits=m  TranslationThetaOffset=0  TranslationThetaOffsetUnits=deg  RotationMethod=ArbitraryAxis  RotationAngleUnits=rad  RotationStandardAxis=+Z  RotationAngle=smiData.RigidTransform(12).angle  RotationArbitraryAxis=smiData.RigidTransform(12).axis  FollAlignAxisA=+X  BaseAlignAxisA=+Y  FollAlignAxisB=+Y  BaseAlignAxisB=+Z  RotationSequenceAxes=FollowerAxes  RotationSequence=XYX  RotationSequenceAngles=[0 0 0]  RotationSequenceAnglesUnits=deg  RotationMatrix=[1 0 0; 0 1 0; 0 0 1]  Quaternion=[1 0 0 0]
  Transform1 : sm_lib/Frames and Transforms/Rigid Transform  TranslationMethod=Cartesian  TranslationStandardOffset=0  TranslationLengthUnit=mm  TranslationStandardAxis=+Z  TranslationCartesianOffset=smiData.RigidTransform(33).translation  TranslationROffset=0  TranslationROffsetUnits=m  TranslationZOffset=0  TranslationZOffsetUnits=m  TranslationThetaOffset=0  TranslationThetaOffsetUnits=deg  RotationMethod=ArbitraryAxis  RotationAngleUnits=rad  RotationStandardAxis=+Z  RotationAngle=smiData.RigidTransform(33).angle  RotationArbitraryAxis=smiData.RigidTransform(33).axis  FollAlignAxisA=+X  BaseAlignAxisA=+Y  FollAlignAxisB=+Y  BaseAlignAxisB=+Z  RotationSequenceAxes=FollowerAxes  RotationSequence=XYX  RotationSequenceAngles=[0 0 0]  RotationSequenceAnglesUnits=deg  RotationMatrix=[1 0 0; 0 1 0; 0 0 1]  Quaternion=[1 0 0 0]
  Transform2 : sm_lib/Frames and Transforms/Rigid Transform  TranslationMethod=Cartesian  TranslationStandardOffset=0  TranslationLengthUnit=mm  TranslationStandardAxis=+Z  TranslationCartesianOffset=smiData.RigidTransform(41).translation  TranslationROffset=0  TranslationROffsetUnits=m  TranslationZOffset=0  TranslationZOffsetUnits=m  TranslationThetaOffset=0  TranslationThetaOffsetUnits=deg  RotationMethod=ArbitraryAxis  RotationAngleUnits=rad  RotationStandardAxis=+Z  RotationAngle=smiData.RigidTransform(41).angle  RotationArbitraryAxis=smiData.RigidTransform(41).axis  FollAlignAxisA=+X  BaseAlignAxisA=+Y  FollAlignAxisB=+Y  BaseAlignAxisB=+Z  RotationSequenceAxes=FollowerAxes  RotationSequence=XYX  RotationSequenceAngles=[0 0 0]  RotationSequenceAnglesUnits=deg  RotationMatrix=[1 0 0; 0 1 0; 0 0 1]  Quaternion=[1 0 0 0]
  F : PMIOPort  Side=Left
  Target : PMIOPort  Port=2  Side=Left
  F2 : PMIOPort  Port=3  Side=Left
  F1 : PMIOPort  Port=4  Side=Right
  connections:
  ReferenceFrame/RConn1 -- Transform1/LConn1 -- Transform2/LConn1 -- Transform/LConn1 -- Target/RConn1 -- Solid/RConn1
  Transform/RConn1 -- F/RConn1
  Transform1/RConn1 -- F1/RConn1
  Transform2/RConn1 -- F2/RConn1

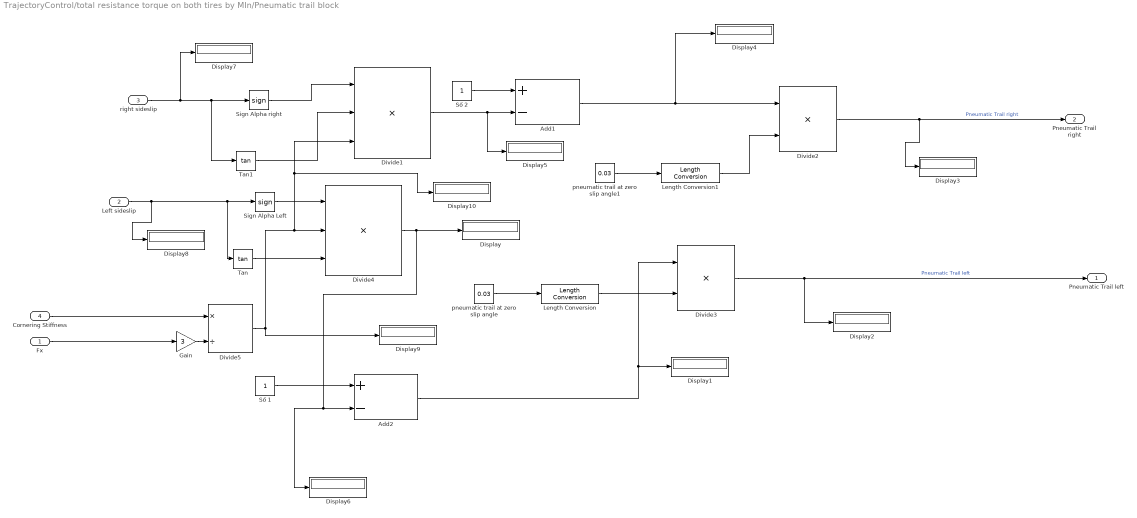
== system TrajectoryControl/total resistance torque on both tires by MIn/Pneumatic trail block ==
  Fx : Inport
  Left sideslip : Inport  Port=2
  right sideslip : Inport  Port=3
  Cornering Stiffness : Inport  Port=4
  Add1 : Sum  Inputs=+-
  Add2 : Sum  Inputs=+-
  Display{,1..10} (11 alike) : Display
  Divide1 : Product  Inputs=***
  Divide2 : Product  Inputs=**
  Divide3 : Product  Inputs=**
  Divide4 : Product  Inputs=***
  Divide5 : Product  Inputs=*/
  Gain : Gain  Gain=3
  Length Conversion : aerolibconvert2/Length Conversion  IU=m  OU=m
  Length Conversion1 : aerolibconvert2/Length Conversion  IU=m  OU=m
  Sign Alpha Left : Signum
  Sign Alpha right : Signum
  Số 1 : Constant
  Số 2 : Constant
  Tan : Trigonometry  Operator=tan
  Tan1 : Trigonometry  Operator=tan
  pneumatic trail at zero slip angle : Constant  Value=0.03
  pneumatic trail at zero slip angle1 : Constant  Value=0.03
  Pneumatic Trail left : Outport
  Pneumatic Trail right : Outport  Port=2
  wires:
  Số 1/1 -> Add2/1
  Divide4/1 -> Display/1, Display6/1, Add2/2
  Divide5/1 -> Display10/1, Divide1/3, Divide4/2, Display9/1
  Tan/1 -> Divide4/3
  pneumatic trail at zero slip angle/1 -> Length Conversion/1
  Gain/1 -> Divide5/2
  Add2/1 -> Display1/1, Divide3/1
  Left sideslip/1 -> Display8/1, Tan/1, Sign Alpha Left/1
  Divide3/1 -> Display2/1, Pneumatic Trail left/1  "Pneumatic Trail left"
  right sideslip/1 -> Display7/1, Tan1/1, Sign Alpha right/1
  Fx/1 -> Gain/1
  Cornering Stiffness/1 -> Divide5/1
  Length Conversion/1 -> Divide3/2
  Sign Alpha Left/1 -> Divide4/1
  Sign Alpha right/1 -> Divide1/1
  Tan1/1 -> Divide1/2
  Divide1/1 -> Display5/1, Add1/2
  Số 2/1 -> Add1/1
  pneumatic trail at zero slip angle1/1 -> Length Conversion1/1
  Add1/1 -> Display4/1, Divide2/1
  Length Conversion1/1 -> Divide2/2
  Divide2/1 -> Display3/1, Pneumatic Trail right/1  "Pneumatic Trail right"
